simulink model "UserInterfaceApplication"  (Simulink 8.3)
settings: Solver=FixedStepDiscrete  StartTime=0.0  StopTime=inf  RelTol=1e-3
undefined symbols (not defined in the file or in its folder): serial
libraries: instrumentlib x3
settings Model: Creator=paddockt  LastModifiedBy=paddockt
settings DataIOCC: SignalLoggingSaveFormat=Dataset
settings DebuggingCC: UnderspecifiedInitializationDetection=Simplified  StateNameClashWarn=none
settings GRTTargetCC: CombineOutputUpdateFcns=on  GRTInterface=off

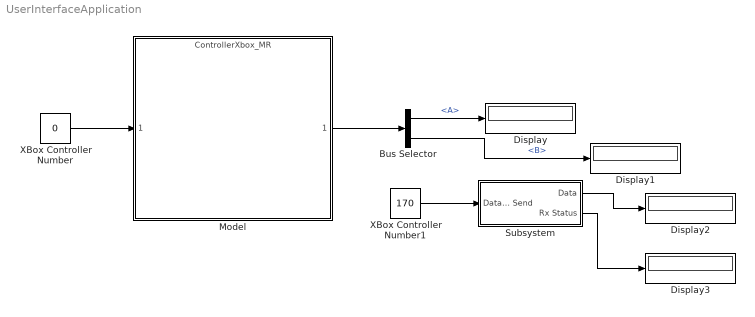
== system UserInterfaceApplication ==
  Bus Selector : BusSelector  OutputSignals=A,B
  Display{,1..3} (4 alike) : Display
  Model : ModelReference  ModelNameDialog=ControllerXbox_MR.mdl  ModelReferenceVersion=1.13  CopyOfModelName=ControllerXbox_MR.mdl  DefaultDataLogging=on
  Subsystem : Subsystem
  XBox Controller Number : Constant  Value=0
  XBox Controller Number1 : Constant  Value=170
  wires:
  XBox Controller Number/1 -> Model/1
  Model/1 -> Bus Selector/1
  Bus Selector/1 -> Display/1  "<A>"
  Bus Selector/2 -> Display1/1  "<B>"
  Subsystem/1(Data) -> Display2/1
  Subsystem/2(Rx Status) -> Display3/1
  XBox Controller Number1/1 -> Subsystem/1(Data To Send)

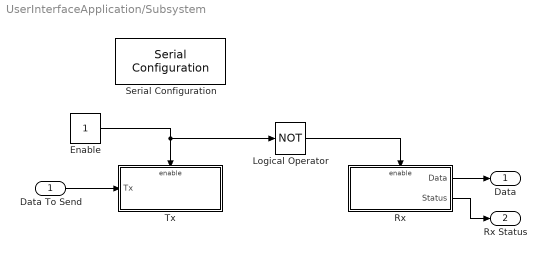
== system UserInterfaceApplication/Subsystem ==
  Data To Send : Inport
  Enable : Constant
  Logical Operator : Logic  Operator=NOT  AllPortsSameDT=off  OutDataTypeStr=boolean
  Rx : Subsystem  TreatAsAtomicUnit=on
  Serial Configuration : instrumentlib/Serial Configuration  Priority=-200000  ComPortMenu=COM4  ComPort=COM5  ObjConstructor=serial('COM5');  BaudRate=9600  DataBits=8  Parity=none  StopBits=1  FlowControl=none  Timeout=3  ByteOrder=LittleEndian
  Tx : Subsystem  TreatAsAtomicUnit=on
  Data : Outport
  Rx Status : Outport  Port=2
  wires:
  Data To Send/1 -> Tx/1(Tx)
  Rx/1(Data) -> Data/1
  Enable/1 -> Logical Operator/1, Tx/Enable
  Logical Operator/1 -> Rx/Enable
  Rx/2(Status) -> Rx Status/1

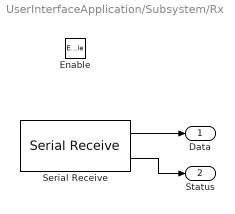
== system UserInterfaceApplication/Subsystem/Rx ==
  Enable : EnablePort
  Serial Receive : instrumentlib/Serial Receive  ComPortMenu=COM5  ComPort=COM5  ObjConstructor=serial('COM5');  Terminator=<none>  DataSize=1  DataType=uint8  EnableBlockingMode=off  ActionDataUnavailable=Output custom value  CustomValue=-1  SampleTime=.5
  Data : Outport
  Status : Outport  Port=2
  wires:
  Serial Receive/1 -> Data/1
  Serial Receive/2 -> Status/1

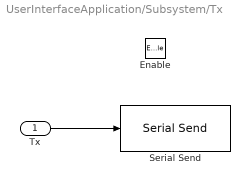
== system UserInterfaceApplication/Subsystem/Tx ==
  Tx : Inport
  Enable : EnablePort
  Serial Send : instrumentlib/Serial Send  ComPortMenu=COM5  ComPort=COM5  ObjConstructor=serial('COM5');  Terminator=<none>  EnableBlockingMode=on
  wires:
  Tx/1 -> Serial Send/1
